simulink model "simulink2"  (R2024a)
settings: Solver=VariableStepAuto  StartTime=0.0  StopTime=10.0  RelTol=1e-3
settings Model: Creator=parsaofrivia  LastModifiedBy=parsaofrivia

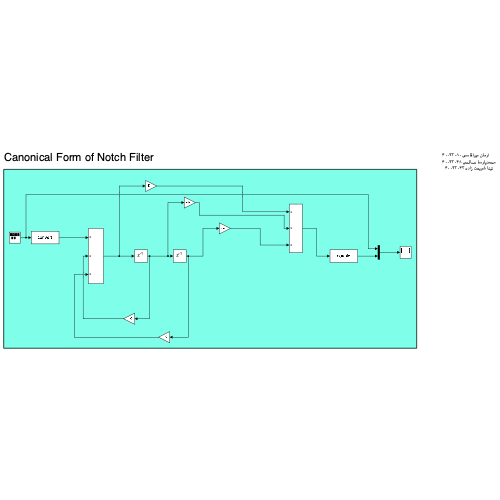
[thumbnail: Simulink's stored preview of the top-level diagram]
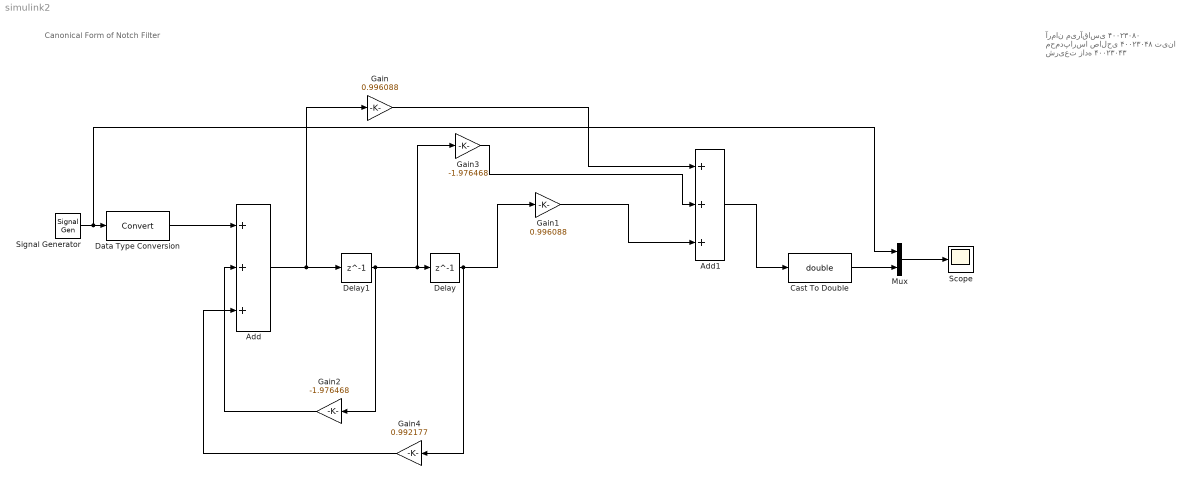
== system simulink2 ==
  note: آرمان میرآقاسی ۴۰۰۲۳۰۸۰
      | محمدپارسا صالحی ۴۰۰۲۳۰۴۸
      | تینا شریعت زاده ۴۰۰۲۳۰۴۳
  note: Canonical Form of Notch Filter
  Add : Sum  Inputs=+++
  Add1 : Sum  Inputs=+++
  Cast To Double : DataTypeConversion  OutDataTypeStr=double  SaturateOnIntegerOverflow=off  RndMeth=Floor
  Data Type Conversion : DataTypeConversion  SaturateOnIntegerOverflow=off  RndMeth=Floor
  Delay : Delay  DelayLength=1  InitialCondition=0
  Delay1 : Delay  DelayLength=1  InitialCondition=0
  Gain : Gain  Gain=0.996088
  Gain1 : Gain  Gain=0.996088
  Gain2 : Gain  Gain=-1.976468
  Gain3 : Gain  Gain=-1.976468
  Gain4 : Gain  Gain=0.992177
  Mux : Mux  Inputs=2
  Scope : Scope
  Signal Generator : SignalGenerator  Frequency=400  Units=rad/sec
  wires:
  Cast To Double/1 -> Mux/2
  Add/1 -> Delay1/1, Gain/1
  Add1/1 -> Cast To Double/1
  Gain2/1 -> Add/2
  Delay1/1 -> Gain2/1, Gain3/1, Delay/1
  Gain1/1 -> Add1/3
  Data Type Conversion/1 -> Add/1
  Gain3/1 -> Add1/2
  Delay/1 -> Gain4/1, Gain1/1
  Gain/1 -> Add1/1
  Mux/1 -> Scope/1
  Signal Generator/1 -> Mux/1, Data Type Conversion/1
  Gain4/1 -> Add/3
